simulink model "Ejemplo7_2_Kuo"  (Simulink 5.0)
settings: Solver=ode45  StartTime=0.0  StopTime=200  RelTol=1e-3
undefined symbols (not defined in the file or in its folder): k
libraries: simulink x2
settings Model: LastModifiedBy=gaby

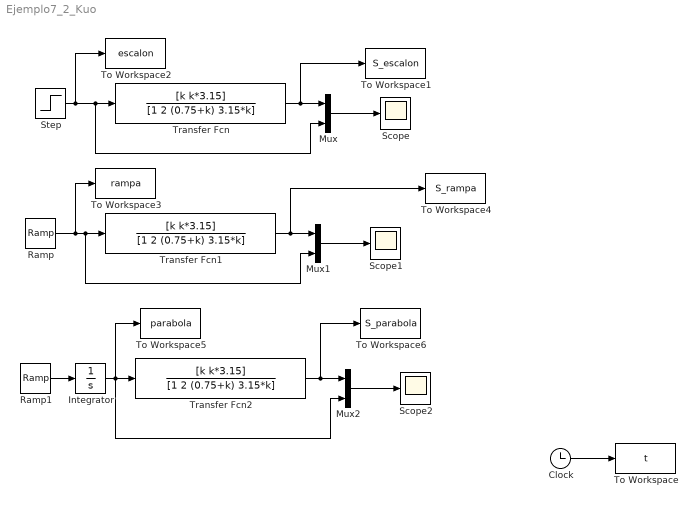
== system Ejemplo7_2_Kuo ==
  Clock : Clock
      settings: Decimation=10
  Integrator : Integrator
  Mux : Mux  Inputs=2
  Mux1 : Mux  Inputs=2
  Mux2 : Mux  Inputs=2
  Ramp : simulink/Sources/Ramp  slope=1  start=0  X0=0
  Ramp1 : simulink/Sources/Ramp  slope=0.5  start=0  X0=0
  Scope : Scope
  Scope1 : Scope
  Scope2 : Scope
      settings: SaveName=ScopeData2
  Step : Step  SampleTime=0
  To Workspace : ToWorkspace  VariableName=t  SampleTime=-1  SaveFormat=Array
  To Workspace1 : ToWorkspace  VariableName=S_escalon  SampleTime=-1  SaveFormat=Array
  To Workspace2 : ToWorkspace  VariableName=escalon  SampleTime=-1  SaveFormat=Array
  To Workspace3 : ToWorkspace  VariableName=rampa  SampleTime=-1  SaveFormat=Array
  To Workspace4 : ToWorkspace  VariableName=S_rampa  SampleTime=-1  SaveFormat=Array
  To Workspace5 : ToWorkspace  VariableName=parabola  SampleTime=-1  SaveFormat=Array
  To Workspace6 : ToWorkspace  VariableName=S_parabola  SampleTime=-1  SaveFormat=Array
  Transfer Fcn : TransferFcn  Numerator=[k k*3.15]  Denominator=[1 2 (0.75+k) 3.15*k]
  Transfer Fcn1 : TransferFcn  Numerator=[k k*3.15]  Denominator=[1 2 (0.75+k) 3.15*k]
  Transfer Fcn2 : TransferFcn  Numerator=[k k*3.15]  Denominator=[1 2 (0.75+k) 3.15*k]
  wires:
  Step/1 -> Transfer Fcn/1, Mux/2, To Workspace2/1
  Transfer Fcn/1 -> Mux/1, To Workspace1/1
  Mux/1 -> Scope/1
  Ramp/1 -> Mux1/2, Transfer Fcn1/1, To Workspace3/1
  Transfer Fcn1/1 -> Mux1/1, To Workspace4/1
  Mux1/1 -> Scope1/1
  Transfer Fcn2/1 -> Mux2/1, To Workspace6/1
  Mux2/1 -> Scope2/1
  Ramp1/1 -> Integrator/1
  Integrator/1 -> Transfer Fcn2/1, Mux2/2, To Workspace5/1
  Clock/1 -> To Workspace/1
